simulink subsystem "SimOut"  (R2024b)
settings: Solver=VariableStepAuto  StartTime=0.0  StopTime=10.0  RelTol=1e-3
undefined symbols (not defined in the file): SimIn
settings Model: Creator=macheson  LastModifiedBy=macheson

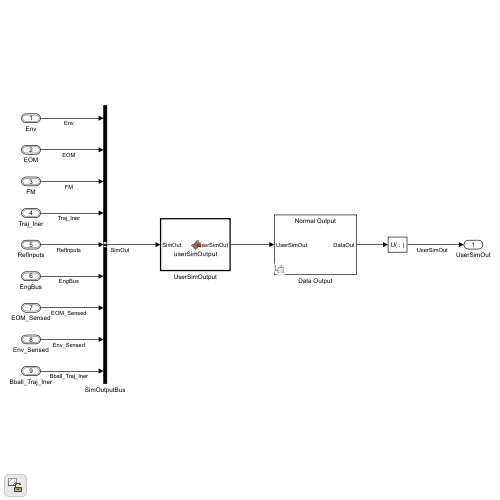
[thumbnail: Simulink's stored preview of the top-level diagram]
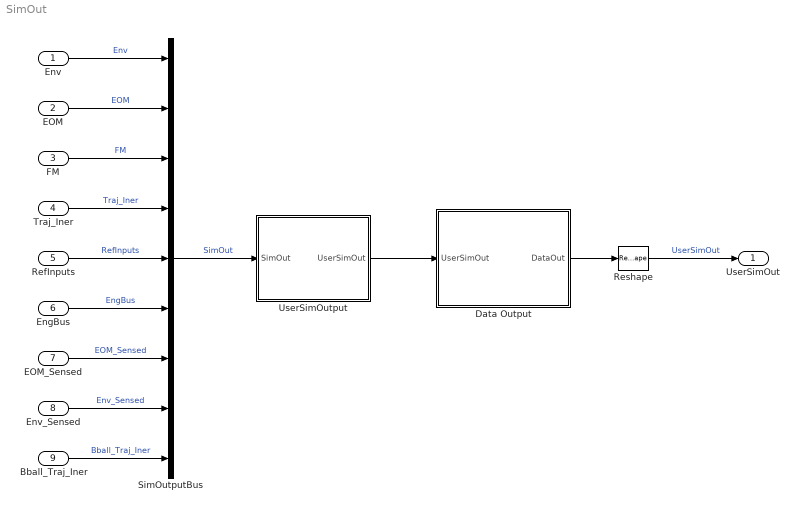
== system SimOut ==
  Env : Inport  OutDataTypeStr=Bus: BUS_ENVIRONMENT
  EOM : Inport  Port=2  OutDataTypeStr=Bus: BUS_EOM
  FM : Inport  Port=3  OutDataTypeStr=Bus: BUS_FORCE_MOMENT
  Traj_Iner : Inport  Port=4  OutDataTypeStr=Bus: BUS_REF_INPUT_INER
  RefInputs : Inport  Port=5  OutDataTypeStr=Bus: BUS_REF_INPUT
  EngBus : Inport  Port=6  OutDataTypeStr=Bus: BUS_PROP_CMD
  EOM_Sensed : Inport  Port=7  OutDataTypeStr=Bus: BUS_EOM
  Env_Sensed : Inport  Port=8  OutDataTypeStr=Bus: BUS_ENVIRONMENT
  Bball_Traj_Iner : Inport  Port=9  OutDataTypeStr=Bus: BUS_REF_INPUT_INER
  Data Output : Subsystem  Variant=on  VariantControl=VectorizeOutput
  Reshape : Reshape
  SimOutputBus : BusCreator  Inputs=9  OutDataTypeStr=Bus: BUS_SIM_OUT  NonVirtualBus=on
  UserSimOutput : MATLAB Function  TreatAsAtomicUnit=on
  UserSimOut : Outport
  wires:
  SimOutputBus/1 -> UserSimOutput/1(SimOut)  "SimOut"
  EOM_Sensed/1 -> SimOutputBus/7  "EOM_Sensed"
  Env_Sensed/1 -> SimOutputBus/8  "Env_Sensed"
  EngBus/1 -> SimOutputBus/6  "EngBus"
  RefInputs/1 -> SimOutputBus/5  "RefInputs"
  Env/1 -> SimOutputBus/1  "Env"
  EOM/1 -> SimOutputBus/2  "EOM"
  FM/1 -> SimOutputBus/3  "FM"
  Traj_Iner/1 -> SimOutputBus/4  "Traj_Iner"
  UserSimOutput/1(UserSimOut) -> Data Output/1(UserSimOut)
  Data Output/1(DataOut) -> Reshape/1
  Reshape/1 -> UserSimOut/1  "UserSimOut"
  Bball_Traj_Iner/1 -> SimOutputBus/9  "Bball_Traj_Iner"

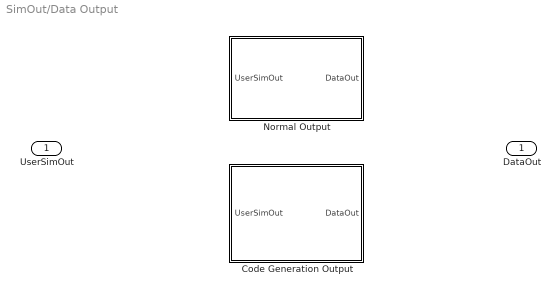
== system SimOut/Data Output ==
  UserSimOut : Inport
  Code Generation Output : MATLAB Function  TreatAsAtomicUnit=on  VariantControl=GVS_DATAOUT_TYPE_CODEGEN  mask{lengthUserOut=SimIn.lengthUserOut}
      mask prompts: lengthUserOut "Num Elements UserOut"
  Normal Output : Subsystem  VariantControl=GVS_DATAOUT_TYPE_NORMAL
  DataOut : Outport

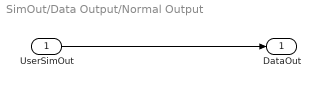
== system SimOut/Data Output/Normal Output ==
  UserSimOut : Inport
  DataOut : Outport
  wires:
  UserSimOut/1 -> DataOut/1

== matlab function SimOut/UserSimOutput ==
  data: SimOut input Bus: BUS_SIM_OUT; UserSimOut output Bus: BUS_USER_SIM_OUT
function UserSimOut  = userSimOutput(SimOut)

  UserSimOut = mapToUserSimOut(SimOut);

end

== matlab function SimOut/Data Output/Code Generation Output ==
  data: UserSimOut input; DataOut output; lengthUserOut parameter
function DataOut  = vectorizeOutput(UserSimOut, lengthUserOut)

  DataOut = zeros(lengthUserOut, 1);

  DataOut(1:lengthUserOut,1) = vectorizeUserSimOut(UserSimOut, lengthUserOut);

end
